simulink model "first_sim"  (R2020b)
settings: Solver=VariableStepAuto  StartTime=0.0  StopTime=10.0  MaxStep=0.01  RelTol=1e-3
settings Model: Creator=shrin  LastModifiedBy=shrin

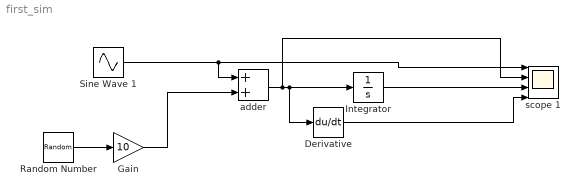
== system first_sim ==
  Derivative : Derivative
  Gain : Gain  Gain=10
  Integrator : Integrator
  Random Number : RandomNumber  SampleTime=0.1
  Sine Wave 1 : Sin  SampleTime=0
  adder : Sum
  scope 1 : Scope  NumInputPorts=4
  wires:
  Sine Wave 1/1 -> scope 1/1, adder/1
  adder/1 -> scope 1/2, Derivative/1, Integrator/1
  Integrator/1 -> scope 1/3
  Random Number/1 -> Gain/1
  Gain/1 -> adder/2
  Derivative/1 -> scope 1/4
